simulink model "ThreePhaseFWCONThyristor"  (Simulink 7.5)
settings: Solver=ode23tb  StartTime=0.0  StopTime=0.5  RelTol=1e-3
libraries: powerlib x21
settings Model: Creator=ninad gaikawad  LastModifiedBy=ninad gaikawad
settings SolverCC: ZeroCrossAlgorithm=Adaptive

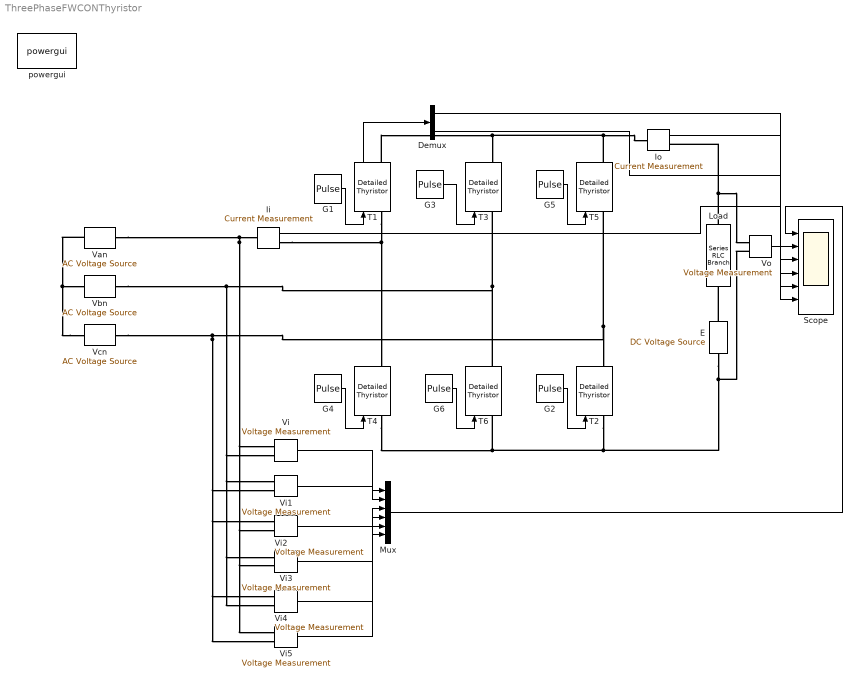
== system ThreePhaseFWCONThyristor ==
  Demux : Demux  Outputs=2
  E : powerlib/Electrical Sources/DC Voltage Source  DialogController=POWERSYS.PowerSysDialog  SystemSampleTime=-1  Amplitude=300  Measurements=None
  G1 : DiscretePulseGenerator  PulseType=Time based  Amplitude=1  Period=20*10^(-3)  PulseWidth=5  PhaseDelay=1/600+1/120  SampleTime=1
  G2 : DiscretePulseGenerator  PulseType=Time based  Amplitude=1  Period=20*10^(-3)  PulseWidth=5  PhaseDelay=1/600+1/120+1/300  SampleTime=1  VectorParams1D=off
  G3 : DiscretePulseGenerator  PulseType=Time based  Amplitude=1  Period=20*10^(-3)  PulseWidth=5  PhaseDelay=1/600+1/120+2/300  SampleTime=1
  G4 : DiscretePulseGenerator  PulseType=Time based  Amplitude=1  Period=20*10^(-3)  PulseWidth=5  PhaseDelay=1/600+1/120+3/300  SampleTime=1
  G5 : DiscretePulseGenerator  PulseType=Time based  Amplitude=1  Period=20*10^(-3)  PulseWidth=5  PhaseDelay=1/600+1/120+4/300  SampleTime=1
  G6 : DiscretePulseGenerator  PulseType=Time based  Amplitude=1  Period=20*10^(-3)  PulseWidth=5  PhaseDelay=1/600+1/120+5/300  SampleTime=1
  Ii : powerlib/Measurements/Current Measurement  DialogController=POWERSYS.PowerSysDialog  SystemSampleTime=-1  PhasorSimulation=off  OutputType=Complex  PSBequivalent=0
  Io : powerlib/Measurements/Current Measurement  DialogController=POWERSYS.PowerSysDialog  SystemSampleTime=-1  PhasorSimulation=off  OutputType=Complex  PSBequivalent=0
  Load : powerlib/Elements/Series RLC Branch  DialogController=POWERSYS.PowerSysDialog  PhysicalDomain=powersysdomain  SubClassName=unknown  LeftPortType=p1  RightPortType=p1  LConnTagsString=__new0  RConnTagsString=__new0  BranchType=RL  Resistance=10  Inductance=6  SetiL0=off  InitialCurrent=0  Capacitance=1e-6  Setx0=off  InitialVoltage=0  Measurements=Branch voltage and current
  Mux : Mux  Inputs=6
  Scope : Scope  NumInputPorts=6
      settings: YMin=-5~-5~-5~-5~-5~-5  YMax=5~5~5~5~5~5
  T{1..6} (6 alike) : powerlib/Power Electronics/Detailed Thyristor  DialogController=POWERSYS.PowerSysDialog  SystemSampleTime=-1  Ron=0.001  Lon=1e-3  Vf=0.8  IL=0.1  Tq=100e-6  IC=0  Rs=500  Cs=250e-9  Measurements=on
  Van : powerlib/Electrical Sources/AC Voltage Source  DialogController=POWERSYS.PowerSysDialog  SystemSampleTime=-1  Amplitude=230  Phase=0  Frequency=50  SampleTime=0  Measurements=None
  Vbn : powerlib/Electrical Sources/AC Voltage Source  DialogController=POWERSYS.PowerSysDialog  SystemSampleTime=-1  Amplitude=230  Phase=-120  Frequency=50  SampleTime=0  Measurements=None
  Vcn : powerlib/Electrical Sources/AC Voltage Source  DialogController=POWERSYS.PowerSysDialog  SystemSampleTime=-1  Amplitude=230  Phase=120  Frequency=50  SampleTime=0  Measurements=None
  Vi{,1..5} (6 alike) : powerlib/Measurements/Voltage Measurement  DialogController=POWERSYS.PowerSysDialog  SystemSampleTime=-1  PhasorSimulation=off  OutputType=Complex  PSBequivalent=0
  Vo : powerlib/Measurements/Voltage Measurement  DialogController=POWERSYS.PowerSysDialog  SystemSampleTime=-1  PhasorSimulation=off  OutputType=Complex  PSBequivalent=0
  powergui : powerlib/powergui  Priority=1  SystemSampleTime=-1  SimulationMode=Continuous  SampleTime=50e-6  frequency=60  SPID=off  DisableSnubberDevices=off  DisableRonSwitches=off  DisableVfSwitches=off  SwTol=0  Interpol=off  frequencyindice=50  echomessages=off  HookPort=off  DisplayEquations=off  FunctionMessages=off  EnableUseOfTLC=off  x0status=blocks  RestoreLinks=warning  ResistiveCurrentMeasurement=off  Ylog=off  Xlog=on  ShowGrid=off  save=off  variable=ZData  ZoomFFT=off  StartTime=0.0  cycles=1  DisplayStyle=1  FreqAxis=off  MaxFrequency=1000  frequencyindicesteady=1  display=off  methode=off
  wires:
  Vi/1 -> Mux/1
  Vi1/1 -> Mux/2
  Vi2/1 -> Mux/3
  G1/1 -> T1/1
  G3/1 -> T3/1
  G5/1 -> T5/1
  G2/1 -> T2/1
  G6/1 -> T6/1
  G4/1 -> T4/1
  Vo/1 -> Scope/2
  Vi3/1 -> Mux/4
  Vi4/1 -> Mux/5
  Vi5/1 -> Mux/6
  T1/1 -> Demux/1
  Mux/1 -> Scope/1
  Ii/1 -> Scope/3
  Io/1 -> Scope/4
  Demux/1 -> Scope/6
  Demux/2 -> Scope/5
  connections:
  T1/LConn1 -- T4/RConn1 -- Ii/RConn1
  Io/LConn1 -- T5/RConn1 -- T1/RConn1 -- T3/RConn1
  Van/RConn1 -- Ii/LConn1 -- Vi3/LConn2 -- Vi5/LConn1 -- Vi/LConn1 -- Vi2/LConn2
  Vbn/RConn1 -- Vi1/LConn1 -- Vi/LConn2 -- Vi3/LConn1 -- Vi4/LConn2 -- T6/RConn1 -- T3/LConn1
  T5/LConn1 -- T2/RConn1 -- Vcn/RConn1 -- Vi2/LConn1 -- Vi1/LConn2 -- Vi4/LConn1 -- Vi5/LConn2
  Vo/LConn2 -- T2/LConn1 -- T4/LConn1 -- T6/LConn1 -- E/RConn1
  Load/LConn1 -- Io/RConn1 -- Vo/LConn1
  Vcn/LConn1 -- Vbn/LConn1 -- Van/LConn1
  E/LConn1 -- Load/RConn1
